simulink model "pid"  (R2019b)
settings: Solver=VariableStepAuto  StartTime=0.0  StopTime=10.0  RelTol=1e-3
settings Model: Creator=marci  LastModifiedBy=marci

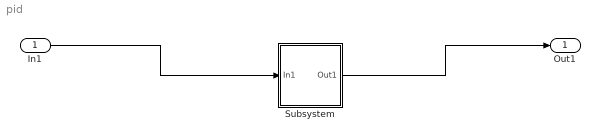
== system pid ==
  In1 : Inport
  Subsystem : Subsystem  mask{P=0, I=0, D=0}
  Out1 : Outport
  wires:
  In1/1 -> Subsystem/1(In1)
  Subsystem/1(Out1) -> Out1/1

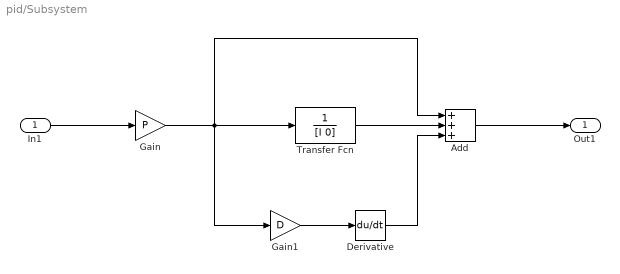
== system pid/Subsystem ==
  In1 : Inport
  Add : Sum  Inputs=+++
  Derivative : Derivative
  Gain : Gain  Gain=P
  Gain1 : Gain  Gain=D
  Transfer Fcn : TransferFcn  Denominator=[I 0]
  Out1 : Outport
  wires:
  Gain/1 -> Add/1, Transfer Fcn/1, Gain1/1
  Transfer Fcn/1 -> Add/2
  Derivative/1 -> Add/3
  In1/1 -> Gain/1
  Gain1/1 -> Derivative/1
  Add/1 -> Out1/1
